simulink model "ModelPNG"  (R2023b)
settings: Solver=VariableStepAuto  StartTime=0.0  StopTime=60  RelTol=1e-3
undefined symbols (not defined in the file): D1, D2, I
libraries: matrix_library x4, simulink x3, mcbcontrolslib x2
settings Model: Creator=markzhuang  LastModifiedBy=markzhuang

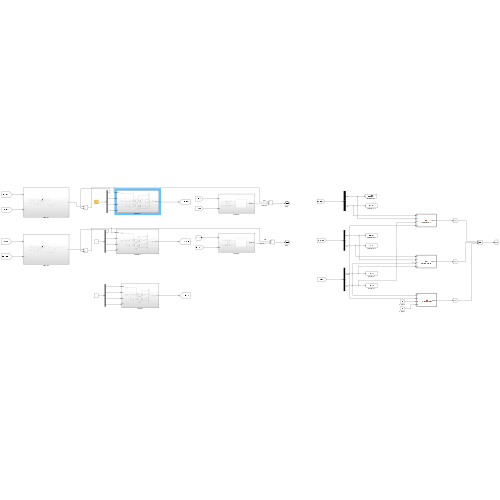
[thumbnail: Simulink's stored preview of the top-level diagram]
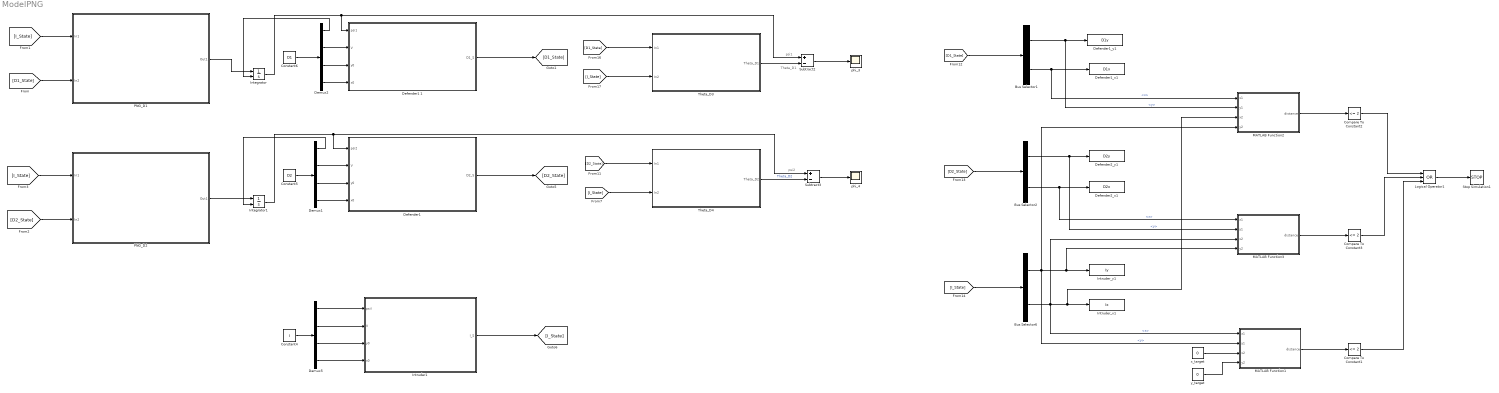
== system ModelPNG ==
  note: Theta_D1
  note: psi1
  note: psi2
  Bus Selector1 : BusSelector  OutputSignals=y,x
  Bus Selector2 : BusSelector  OutputSignals=y,x
  Bus Selector6 : BusSelector  OutputSignals=y,x
  Compare To Constant1 : simulink/Logic and Bit Operations/Compare To Constant  relop=<=  const=2  OutDataTypeStr=boolean
  Compare To Constant2 : simulink/Logic and Bit Operations/Compare To Constant  relop=<=  const=2  OutDataTypeStr=boolean
  Compare To Constant3 : simulink/Logic and Bit Operations/Compare To Constant  relop=<=  const=2  OutDataTypeStr=boolean
  Constant4 : Constant  Value=I  VectorParams1D=off
  Constant5 : Constant  Value=D2  VectorParams1D=off
  Constant6 : Constant  Value=D1  VectorParams1D=off
  Defender1 : Subsystem
  Defender1 1 : Subsystem
  Defender1_x1 : ToWorkspace  VariableName=D1x  SaveFormat=Timeseries  SampleTime=-1
  Defender1_y1 : ToWorkspace  VariableName=D1y  SaveFormat=Timeseries  SampleTime=-1
  Defender2_x1 : ToWorkspace  VariableName=D2x  SaveFormat=Timeseries  SampleTime=-1
  Defender2_y1 : ToWorkspace  VariableName=D2y  SaveFormat=Timeseries  SampleTime=-1
  Demux1 : Demux
  Demux2 : Demux
  Demux5 : Demux
  Integrator : Integrator  InitialConditionSource=external
  Integrator1 : Integrator  InitialConditionSource=external
  Intruder1 : Subsystem
  Intruder_x1 : ToWorkspace  VariableName=Ix  SaveFormat=Timeseries  SampleTime=-1
  Intruder_y1 : ToWorkspace  VariableName=Iy  SaveFormat=Timeseries  SampleTime=-1
  Logical Operator1 : Logic  Operator=OR  Inputs=3  AllPortsSameDT=off  OutDataTypeStr=boolean
  MATLAB Function1 : MATLAB Function  TreatAsAtomicUnit=on
  MATLAB Function2 : MATLAB Function  TreatAsAtomicUnit=on
  MATLAB Function3 : MATLAB Function  TreatAsAtomicUnit=on
  PNG_D1 : Subsystem
  PNG_D2 : Subsystem
  Stop Simulation1 : Stop
  Subtract2 : Sum  Inputs=+-
  Subtract3 : Sum  Inputs=+-
  Theta_D3 : Subsystem
  Theta_D4 : Subsystem
  phi_3 : Scope
  phi_4 : Scope
  x_target : Constant  Value=0
  y_target : Constant  Value=0
  wires:
  [I_State] -> PNG_D1/1(In1)
  Theta_D3/1(Theta_D1) -> Subtract2/2
  [D2_State] -> Bus Selector2/1
  [D1_State] -> PNG_D1/2(In2)
  Logical Operator1/1 -> Stop Simulation1/1
  [D1_State] -> Bus Selector1/1
  Compare To Constant2/1 -> Logical Operator1/1
  MATLAB Function2/1(distance) -> Compare To Constant2/1
  Subtract2/1 -> phi_3/1
  [D2_State] -> Theta_D4/1(In1)
  Subtract3/1 -> phi_4/1
  Intruder1/1(I_S) -> [I_State]
  Defender1 1/1(D1_S) -> [D1_State]
  Constant5/1 -> Demux1/1
  Defender1/1(D2_S) -> [D2_State]
  Bus Selector1/2 -> MATLAB Function2/1(x1), Defender1_x1/1  "<x>"
  [I_State] -> Bus Selector6/1
  Bus Selector2/2 -> MATLAB Function3/1(x1), Defender2_x1/1  "<x>"
  Bus Selector1/1 -> MATLAB Function2/2(y1), Defender1_y1/1  "<y>"
  Theta_D4/1(Theta_D2) -> Subtract3/2  "Theta_D2"
  [D2_State] -> PNG_D2/2(In2)
  Demux1/4 -> Defender1/4(x0)
  Constant6/1 -> Demux2/1
  MATLAB Function3/1(distance) -> Compare To Constant3/1
  [I_State] -> PNG_D2/1(In1)
  Compare To Constant3/1 -> Logical Operator1/2
  [I_State] -> Theta_D4/2(In2)
  [D1_State] -> Theta_D3/1(In1)
  [I_State] -> Theta_D3/2(In2)
  Bus Selector2/1 -> MATLAB Function3/2(y1), Defender2_y1/1  "<y>"
  Constant4/1 -> Demux5/1
  Demux5/1 -> Intruder1/1(psiI)
  Demux5/2 -> Intruder1/2(V)
  Demux5/3 -> Intruder1/3(y0)
  Demux5/4 -> Intruder1/4(x0)
  PNG_D1/1(Out1) -> Integrator/1
  Demux1/3 -> Defender1/3(y0)
  Demux1/2 -> Defender1/2(V)
  Demux2/4 -> Defender1 1/4(x0)
  Demux2/3 -> Defender1 1/3(y0)
  Demux2/2 -> Defender1 1/2(V)
  PNG_D2/1(Out1) -> Integrator1/1
  Integrator/1 -> Defender1 1/1(psi1), Subtract2/1
  Integrator1/1 -> Subtract3/1, Defender1/1(psi2)
  Demux1/1 -> Integrator1/2
  Demux2/1 -> Integrator/2
  y_target/1 -> MATLAB Function1/4(y2)
  Compare To Constant1/1 -> Logical Operator1/3
  MATLAB Function1/1(distance) -> Compare To Constant1/1
  x_target/1 -> MATLAB Function1/3(x2)
  Bus Selector6/2 -> MATLAB Function3/3(x2), MATLAB Function1/1(x1), MATLAB Function2/3(x2), Intruder_x1/1  "<x>"
  Bus Selector6/1 -> MATLAB Function1/2(y1), MATLAB Function2/4(y2), MATLAB Function3/4(y2), Intruder_y1/1  "<y>"

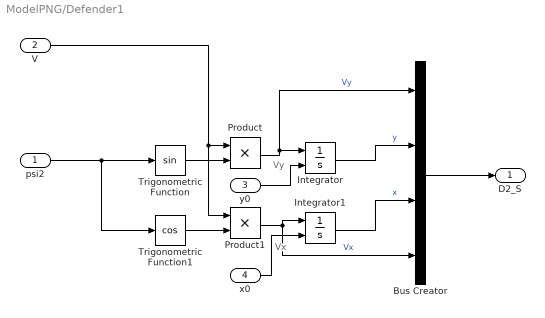
== system ModelPNG/Defender1 ==
  note: Vx
  note: Vy
  psi2 : Inport
  V : Inport  Port=2
  y0 : Inport  Port=3
  x0 : Inport  Port=4
  Bus Creator : BusCreator  Inputs=4
  Integrator : Integrator  InitialConditionSource=external
  Integrator1 : Integrator  InitialConditionSource=external
  Product : Product
  Product1 : Product
  Trigonometric Function : Trigonometry
  Trigonometric Function1 : Trigonometry  Operator=cos
  D2_S : Outport
  wires:
  Trigonometric Function/1 -> Product/2
  Product/1 -> Bus Creator/1, Integrator/1  "Vy"
  psi2/1 -> Trigonometric Function1/1, Trigonometric Function/1
  Product1/1 -> Bus Creator/4, Integrator1/1  "Vx"
  V/1 -> Product1/1, Product/1
  Trigonometric Function1/1 -> Product1/2
  Integrator/1 -> Bus Creator/2  "y"
  Integrator1/1 -> Bus Creator/3  "x"
  y0/1 -> Integrator/2
  x0/1 -> Integrator1/2
  Bus Creator/1 -> D2_S/1

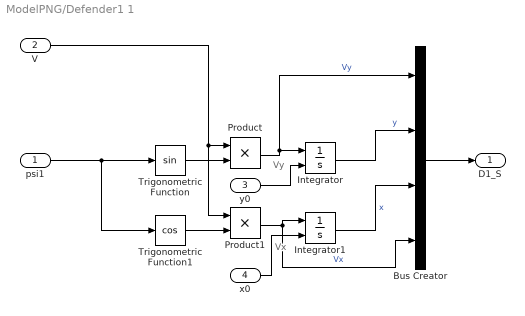
== system ModelPNG/Defender1 1 ==
  note: Vx
  note: Vy
  psi1 : Inport
  V : Inport  Port=2
  y0 : Inport  Port=3
  x0 : Inport  Port=4
  Bus Creator : BusCreator  Inputs=4
  Integrator : Integrator  InitialConditionSource=external
  Integrator1 : Integrator  InitialConditionSource=external
  Product : Product
  Product1 : Product
  Trigonometric Function : Trigonometry
  Trigonometric Function1 : Trigonometry  Operator=cos
  D1_S : Outport
  wires:
  Trigonometric Function/1 -> Product/2
  psi1/1 -> Trigonometric Function1/1, Trigonometric Function/1
  Product1/1 -> Bus Creator/4, Integrator1/1  "Vx"
  V/1 -> Product1/1, Product/1
  Trigonometric Function1/1 -> Product1/2
  y0/1 -> Integrator/2
  x0/1 -> Integrator1/2
  Product/1 -> Bus Creator/1, Integrator/1  "Vy"
  Integrator/1 -> Bus Creator/2  "y"
  Integrator1/1 -> Bus Creator/3  "x"
  Bus Creator/1 -> D1_S/1

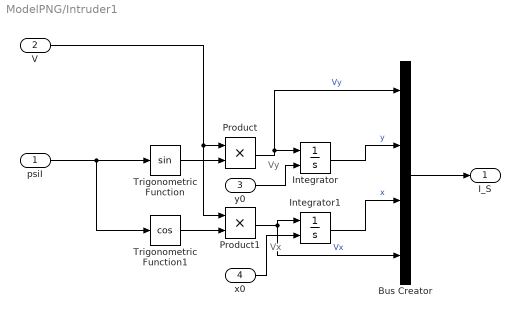
== system ModelPNG/Intruder1 ==
  note: Vx
  note: Vy
  psiI : Inport
  V : Inport  Port=2
  y0 : Inport  Port=3
  x0 : Inport  Port=4
  Bus Creator : BusCreator  Inputs=4
  Integrator : Integrator  InitialConditionSource=external
  Integrator1 : Integrator  InitialConditionSource=external
  Product : Product
  Product1 : Product
  Trigonometric Function : Trigonometry
  Trigonometric Function1 : Trigonometry  Operator=cos
  I_S : Outport
  wires:
  Trigonometric Function/1 -> Product/2
  Product/1 -> Bus Creator/1, Integrator/1  "Vy"
  psiI/1 -> Trigonometric Function1/1, Trigonometric Function/1
  Product1/1 -> Bus Creator/4, Integrator1/1  "Vx"
  V/1 -> Product1/1, Product/1
  Trigonometric Function1/1 -> Product1/2
  Integrator/1 -> Bus Creator/2  "y"
  Integrator1/1 -> Bus Creator/3  "x"
  y0/1 -> Integrator/2
  x0/1 -> Integrator1/2
  Bus Creator/1 -> I_S/1

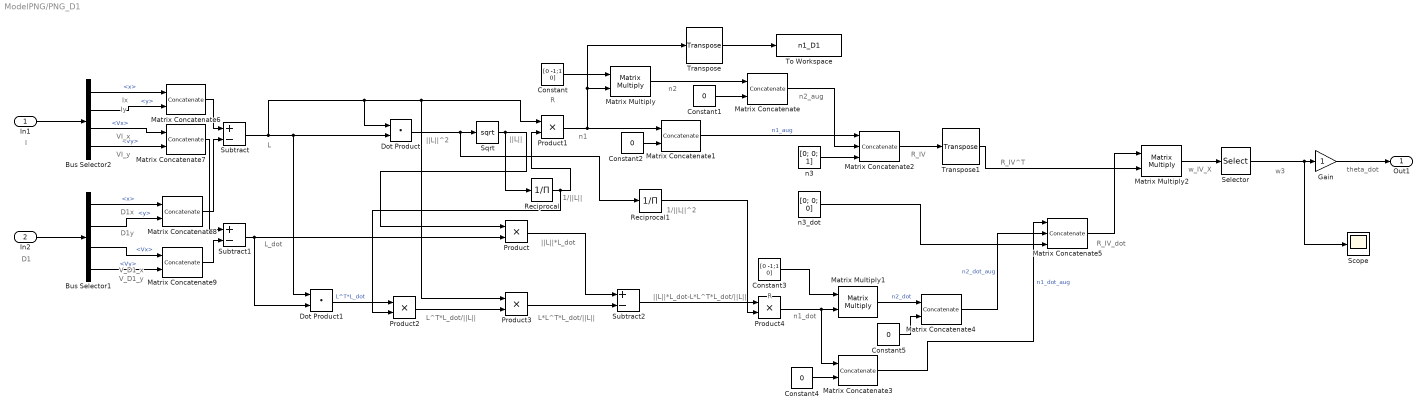
== system ModelPNG/PNG_D1 ==
  note: 1/||L||^2
  note: 1/||L||
  note: R_IV^T
  note: R_IV_dot
  note: R_IV
  note: n2_aug
  note: n2
  note: R
  note: n1_dot
  note: L^T*L_dot/||L||
  note: ||L||*L_dot
  note: n1
  note: ||L||
  note: ||L||^2
  note: L_dot
  note: theta_dot
  note: w3
  note: w_IV_X
  note: VI_y
  note: VI_x
  note: D1
  note: I
  note: Ix
  note: Iy
  note: L
  note: D1y
  note: D1x
  note: V_D1_x
  note: V_D1_y
  note: L*L^T*L_dot/||L||
  note: ||L||*L_dot-L*L^T*L_dot/||L||
  note: R
  In1 : Inport
  In2 : Inport  Port=2
  Bus Selector1 : BusSelector  OutputSignals=x,y,Vx,Vy
  Bus Selector2 : BusSelector  OutputSignals=x,y,Vx,Vy
  Constant : Constant  Value=[0 -1;1 0]  VectorParams1D=off
  Constant{1..2,4..5} (4 alike) : Constant  Value=0  VectorParams1D=off
  Constant3 : Constant  Value=[0 -1;1 0]  VectorParams1D=off
  Dot Product : DotProduct  OutDataTypeStr=Inherit: Inherit via internal rule
  Dot Product1 : DotProduct  OutDataTypeStr=Inherit: Inherit via internal rule
  Gain : Gain
  Matrix Concatenate{,1,3..4,6..9} (8 alike) : Concatenate  Mode=Multidimensional array
  Matrix Concatenate2 : Concatenate  NumInputs=3  Mode=Multidimensional array  ConcatenateDimension=2
  Matrix Concatenate5 : Concatenate  NumInputs=3  Mode=Multidimensional array  ConcatenateDimension=2
  Matrix Multiply : Product  Multiplication=Matrix(*)
  Matrix Multiply1 : Product  Multiplication=Matrix(*)
  Matrix Multiply2 : Product  Multiplication=Matrix(*)
  Product{,1..4} (5 alike) : Product
  Reciprocal : Product  Inputs=/
  Reciprocal1 : Product  Inputs=/
  Scope : Scope
  Selector : Selector  NumberOfDimensions=2  InputPortWidth=3  IndexOptions=Starting index (dialog),Starting index (dialog)  Indices=2,1  OutputSizes=1,1
  Sqrt : Sqrt
  Subtract : Sum  Inputs=+-
  Subtract1 : Sum  Inputs=+-
  Subtract2 : Sum  Inputs=+-
  To Workspace : ToWorkspace  VariableName=n1_D1  SaveFormat=Structure With Time  SampleTime=-1
  Transpose : matrix_library/Transpose
  Transpose1 : matrix_library/Transpose
  n3 : Constant  Value=[0; 0; 1]  VectorParams1D=off
  n3_dot : Constant  Value=[0; 0; 0]  VectorParams1D=off
  Out1 : Outport
  wires:
  In1/1 -> Bus Selector2/1
  In2/1 -> Bus Selector1/1
  Matrix Multiply2/1 -> Selector/1
  Selector/1 -> Scope/1, Gain/1
  Gain/1 -> Out1/1
  Bus Selector2/1 -> Matrix Concatenate6/1  "<x>"
  Bus Selector1/1 -> Matrix Concatenate8/1  "<x>"
  Bus Selector1/3 -> Matrix Concatenate9/1  "<Vx>"
  Bus Selector1/4 -> Matrix Concatenate9/2  "<Vy>"
  Bus Selector2/2 -> Matrix Concatenate6/2  "<y>"
  Bus Selector2/3 -> Matrix Concatenate7/1  "<Vx>"
  Bus Selector2/4 -> Matrix Concatenate7/2  "<Vy>"
  Bus Selector1/2 -> Matrix Concatenate8/2  "<y>"
  Matrix Concatenate8/1 -> Subtract/2
  Matrix Concatenate6/1 -> Subtract/1
  Matrix Concatenate7/1 -> Subtract1/1
  Matrix Concatenate9/1 -> Subtract1/2
  Subtract/1 -> Dot Product1/1, Dot Product/2, Product3/1, Product1/1, Dot Product/1
  Subtract1/1 -> Dot Product1/2, Product/2
  Dot Product/1 -> Reciprocal1/1, Sqrt/1
  Product1/1 -> Matrix Concatenate1/1, Transpose/1, Matrix Multiply/2
  Sqrt/1 -> Reciprocal/1, Product/1
  Product/1 -> Subtract2/1
  Dot Product1/1 -> Product2/1  "L^T*L_dot"
  Product2/1 -> Product3/2
  Product3/1 -> Subtract2/2
  Subtract2/1 -> Product4/1
  Product4/1 -> Matrix Concatenate3/1, Matrix Multiply1/2
  Constant/1 -> Matrix Multiply/1
  Matrix Multiply/1 -> Matrix Concatenate/1
  Constant1/1 -> Matrix Concatenate/2
  Constant2/1 -> Matrix Concatenate1/2
  Matrix Concatenate1/1 -> Matrix Concatenate2/1  "n1_aug"
  Matrix Concatenate/1 -> Matrix Concatenate2/2
  n3/1 -> Matrix Concatenate2/3
  Matrix Concatenate2/1 -> Transpose1/1
  Constant3/1 -> Matrix Multiply1/1
  Matrix Multiply1/1 -> Matrix Concatenate4/1  "n2_dot"
  Constant4/1 -> Matrix Concatenate3/2
  Matrix Concatenate3/1 -> Matrix Concatenate5/1  "n1_dot_aug"
  Constant5/1 -> Matrix Concatenate4/2
  n3_dot/1 -> Matrix Concatenate5/3
  Matrix Concatenate4/1 -> Matrix Concatenate5/2  "n2_dot_aug"
  Matrix Concatenate5/1 -> Matrix Multiply2/1
  Transpose1/1 -> Matrix Multiply2/2
  Reciprocal/1 -> Product2/2, Product1/2
  Reciprocal1/1 -> Product4/2
  Transpose/1 -> To Workspace/1

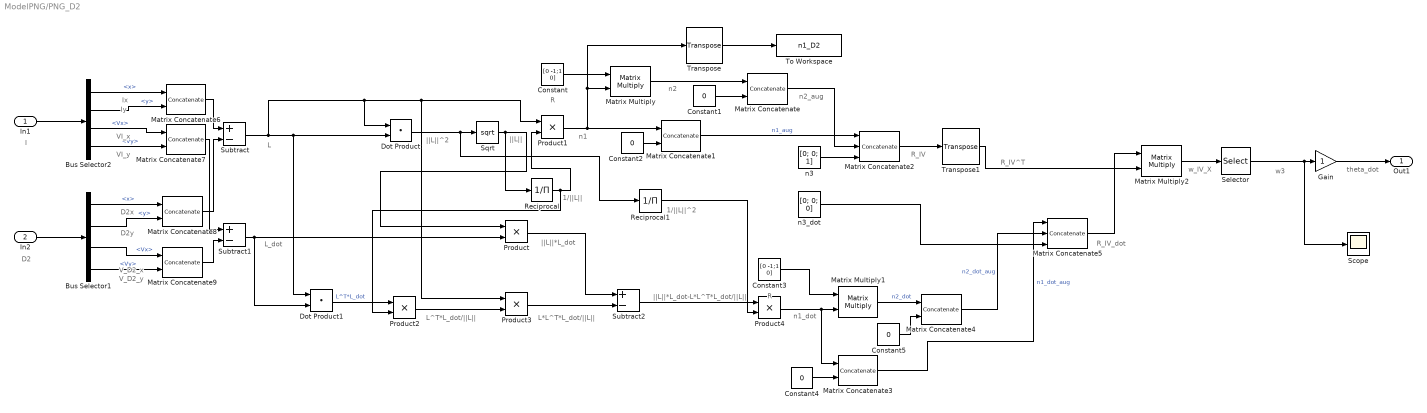
== system ModelPNG/PNG_D2 ==
  note: ||L||*L_dot
  note: V_D2_y
  note: I
  note: ||L||*L_dot-L*L^T*L_dot/||L||
  note: R
  note: VI_x
  note: D2
  note: ||L||^2
  note: Iy
  note: n1_dot
  note: n2_aug
  note: D2y
  note: VI_y
  note: L*L^T*L_dot/||L||
  note: Ix
  note: w3
  note: V_D2_x
  note: D2x
  note: R_IV
  note: L
  note: theta_dot
  note: L_dot
  note: ||L||
  note: n1
  note: R_IV_dot
  note: L^T*L_dot/||L||
  note: w_IV_X
  note: R
  note: n2
  note: R_IV^T
  note: 1/||L||
  note: 1/||L||^2
  In1 : Inport
  In2 : Inport  Port=2
  Bus Selector1 : BusSelector  OutputSignals=x,y,Vx,Vy
  Bus Selector2 : BusSelector  OutputSignals=x,y,Vx,Vy
  Constant : Constant  Value=[0 -1;1 0]  VectorParams1D=off
  Constant{1..2,4..5} (4 alike) : Constant  Value=0  VectorParams1D=off
  Constant3 : Constant  Value=[0 -1;1 0]  VectorParams1D=off
  Dot Product : DotProduct  OutDataTypeStr=Inherit: Inherit via internal rule
  Dot Product1 : DotProduct  OutDataTypeStr=Inherit: Inherit via internal rule
  Gain : Gain
  Matrix Concatenate{,1,3..4,6..9} (8 alike) : Concatenate  Mode=Multidimensional array
  Matrix Concatenate2 : Concatenate  NumInputs=3  Mode=Multidimensional array  ConcatenateDimension=2
  Matrix Concatenate5 : Concatenate  NumInputs=3  Mode=Multidimensional array  ConcatenateDimension=2
  Matrix Multiply : Product  Multiplication=Matrix(*)
  Matrix Multiply1 : Product  Multiplication=Matrix(*)
  Matrix Multiply2 : Product  Multiplication=Matrix(*)
  Product{,1..4} (5 alike) : Product
  Reciprocal : Product  Inputs=/
  Reciprocal1 : Product  Inputs=/
  Scope : Scope
  Selector : Selector  NumberOfDimensions=2  InputPortWidth=3  IndexOptions=Starting index (dialog),Starting index (dialog)  Indices=2,1  OutputSizes=1,1
  Sqrt : Sqrt
  Subtract : Sum  Inputs=+-
  Subtract1 : Sum  Inputs=+-
  Subtract2 : Sum  Inputs=+-
  To Workspace : ToWorkspace  VariableName=n1_D2  SaveFormat=Structure With Time  SampleTime=-1
  Transpose : matrix_library/Transpose
  Transpose1 : matrix_library/Transpose
  n3 : Constant  Value=[0; 0; 1]  VectorParams1D=off
  n3_dot : Constant  Value=[0; 0; 0]  VectorParams1D=off
  Out1 : Outport
  wires:
  Matrix Concatenate5/1 -> Matrix Multiply2/1
  Constant/1 -> Matrix Multiply/1
  Reciprocal1/1 -> Product4/2
  Constant1/1 -> Matrix Concatenate/2
  Product1/1 -> Matrix Concatenate1/1, Transpose/1, Matrix Multiply/2
  Matrix Multiply/1 -> Matrix Concatenate/1
  Matrix Multiply2/1 -> Selector/1
  Bus Selector1/4 -> Matrix Concatenate9/2  "<Vy>"
  Reciprocal/1 -> Product2/2, Product1/2
  Bus Selector2/1 -> Matrix Concatenate6/1  "<x>"
  Product2/1 -> Product3/2
  Matrix Concatenate2/1 -> Transpose1/1
  Subtract1/1 -> Dot Product1/2, Product/2
  Matrix Concatenate4/1 -> Matrix Concatenate5/2  "n2_dot_aug"
  Bus Selector1/1 -> Matrix Concatenate8/1  "<x>"
  n3_dot/1 -> Matrix Concatenate5/3
  Bus Selector1/3 -> Matrix Concatenate9/1  "<Vx>"
  Matrix Concatenate1/1 -> Matrix Concatenate2/1  "n1_aug"
  Matrix Concatenate8/1 -> Subtract/2
  Bus Selector1/2 -> Matrix Concatenate8/2  "<y>"
  Transpose1/1 -> Matrix Multiply2/2
  Dot Product/1 -> Reciprocal1/1, Sqrt/1
  Constant5/1 -> Matrix Concatenate4/2
  Constant4/1 -> Matrix Concatenate3/2
  Matrix Concatenate7/1 -> Subtract1/1
  Product/1 -> Subtract2/1
  Sqrt/1 -> Reciprocal/1, Product/1
  Gain/1 -> Out1/1
  Subtract/1 -> Dot Product1/1, Dot Product/2, Product3/1, Product1/1, Dot Product/1
  Bus Selector2/4 -> Matrix Concatenate7/2  "<Vy>"
  Bus Selector2/2 -> Matrix Concatenate6/2  "<y>"
  Matrix Concatenate6/1 -> Subtract/1
  Matrix Concatenate9/1 -> Subtract1/2
  In2/1 -> Bus Selector1/1
  n3/1 -> Matrix Concatenate2/3
  Bus Selector2/3 -> Matrix Concatenate7/1  "<Vx>"
  Product3/1 -> Subtract2/2
  Constant2/1 -> Matrix Concatenate1/2
  Transpose/1 -> To Workspace/1
  In1/1 -> Bus Selector2/1
  Constant3/1 -> Matrix Multiply1/1
  Matrix Multiply1/1 -> Matrix Concatenate4/1  "n2_dot"
  Product4/1 -> Matrix Concatenate3/1, Matrix Multiply1/2
  Matrix Concatenate3/1 -> Matrix Concatenate5/1  "n1_dot_aug"
  Subtract2/1 -> Product4/1
  Matrix Concatenate/1 -> Matrix Concatenate2/2
  Dot Product1/1 -> Product2/1  "L^T*L_dot"
  Selector/1 -> Scope/1, Gain/1

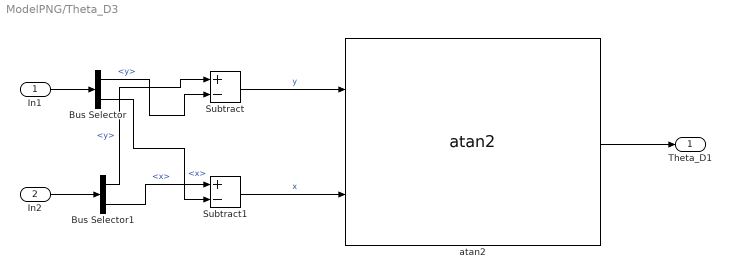
== system ModelPNG/Theta_D3 ==
  In1 : Inport
  In2 : Inport  Port=2
  Bus Selector : BusSelector  OutputSignals=y,x
  Bus Selector1 : BusSelector  OutputSignals=y,x
  Subtract : Sum  Inputs=+-
  Subtract1 : Sum  Inputs=+-
  atan2 : mcbcontrolslib/atan2  ApproximationMethod=None  NumberOfIterations=11  NumberOfDataPoints=16  InterpMethod=Flat  outputUnit=Radians  TableDataTypeStr=Inherit: Inherit via input
      settings: LibrarySourceBlock=mcblib/Controls/Math Transforms/atan2
  Theta_D1 : Outport
  wires:
  In1/1 -> Bus Selector/1
  In2/1 -> Bus Selector1/1
  Bus Selector1/1 -> Subtract/1  "<y>"
  Bus Selector/1 -> Subtract/2  "<y>"
  Bus Selector1/2 -> Subtract1/1  "<x>"
  Bus Selector/2 -> Subtract1/2  "<x>"
  Subtract/1 -> atan2/1  "y"
  Subtract1/1 -> atan2/2  "x"
  atan2/1 -> Theta_D1/1

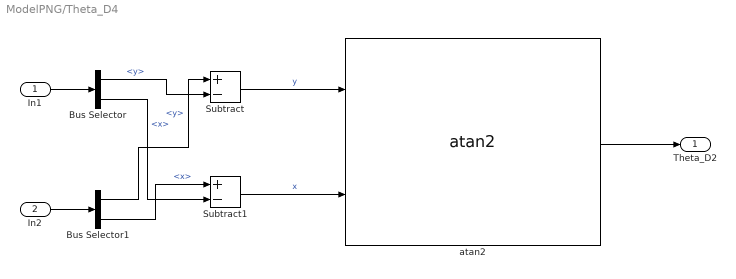
== system ModelPNG/Theta_D4 ==
  In1 : Inport
  In2 : Inport  Port=2
  Bus Selector : BusSelector  OutputSignals=y,x
  Bus Selector1 : BusSelector  OutputSignals=y,x
  Subtract : Sum  Inputs=+-
  Subtract1 : Sum  Inputs=+-
  atan2 : mcbcontrolslib/atan2  ApproximationMethod=None  NumberOfIterations=11  NumberOfDataPoints=16  InterpMethod=Flat  outputUnit=Radians  TableDataTypeStr=Inherit: Inherit via input
      settings: LibrarySourceBlock=mcblib/Controls/Math Transforms/atan2
  Theta_D2 : Outport
  wires:
  In1/1 -> Bus Selector/1
  In2/1 -> Bus Selector1/1
  Bus Selector1/1 -> Subtract/1  "<y>"
  Bus Selector/1 -> Subtract/2  "<y>"
  Bus Selector1/2 -> Subtract1/1  "<x>"
  Bus Selector/2 -> Subtract1/2  "<x>"
  Subtract/1 -> atan2/1  "y"
  Subtract1/1 -> atan2/2  "x"
  atan2/1 -> Theta_D2/1

== matlab function ModelPNG/MATLAB Function1 ==
  data: x1 input; distance output; y1 input; x2 input; y2 input
function distance = calculateDistance(x1, y1, x2, y2)
    distance = sqrt((x2 - x1)^2 + (y2 - y1)^2);
end

== matlab function ModelPNG/MATLAB Function2 ==
  data: x1 input; distance output; y1 input; x2 input; y2 input
function distance = calculateDistance(x1, y1, x2, y2)
    distance = sqrt((x2 - x1)^2 + (y2 - y1)^2);
end

== matlab function ModelPNG/MATLAB Function3 ==
  data: x1 input; distance output; y1 input; x2 input; y2 input
function distance = calculateDistance(x1, y1, x2, y2)
    distance = sqrt((x2 - x1)^2 + (y2 - y1)^2);
end
